simulink model "TPGCI_2"  (R2024a)
settings: Solver=FixedStepDiscrete  StartTime=0.0  StopTime=10.0  FixedStep=2e-5  RelTol=1e-3
undefined symbols (not defined in the file): DiscIntNeverNeededParam
libraries: slpidlib x3
settings Model: Creator=mahes  LastModifiedBy=mahes
settings OptimizationCC: DefaultParameterBehavior=Inlined  UseDivisionForNetSlopeComputation=on  GainParamInheritBuiltInType=on  UseFloatMulNetSlope=on  InlineInvariantSignals=on  PassReuseOutputArgsAs=Individual arguments  ZeroExternalMemoryAtStartup=off  ZeroInternalMemoryAtStartup=off  NoFixptDivByZeroProtection=on  EfficientFloat2IntCast=on  LifeSpan=1  OptimizeBlockOrder=speed  DifferentSizesBufferReuse=on  EfficientTunableParamExpr=on
settings DebuggingCC: ParameterTunabilityLossMsg=error
settings HardwareCC: ProdBitPerPointer=32  ProdBitPerSizeT=32  ProdBitPerPtrDiffT=32  ProdLargestAtomicInteger=Long  ProdLargestAtomicFloat=Double  ProdWordSize=32  ProdLongLongMode=on  ProdHWDeviceType=ARM Compatible->ARM Cortex-M
settings SFSimCC: MATLABDynamicMemAlloc=off
settings RTWCC: Description=Embedded Coder  SystemTargetFile=ert.tlc  TemplateMakefile=ert_default_tmf
settings CodeAppCC: ForceParamTrailComments=on  IgnoreCustomStorageClasses=off  OperatorAnnotations=on  SimulinkDataObjDesc=on  SFDataObjDesc=on  CustomSymbolStrGlobalVar=rt$N$M  CustomSymbolStrType=$N$M  CustomSymbolStrFcn=$N$M$F  CustomSymbolStrMacro=$N$M  InsertBlockDesc=on
settings ERTTargetCC: TargetLangStandard=C99 (ISO)  GenerateSampleERTMain=on  IncludeMdlTerminateFcn=off  CombineSignalStateStructs=on  SupportAbsoluteTime=off  SupportComplex=off  SupportNonInlinedSFcns=on  InlinedParameterPlacement=NonHierarchical  ERTCustomFileTemplate=example_file_process.tlc  ERTFilePackagingFormat=CompactWithDataFile

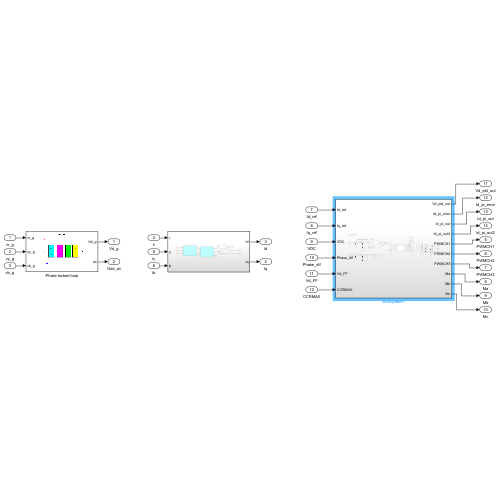
[thumbnail: Simulink's stored preview of the top-level diagram]
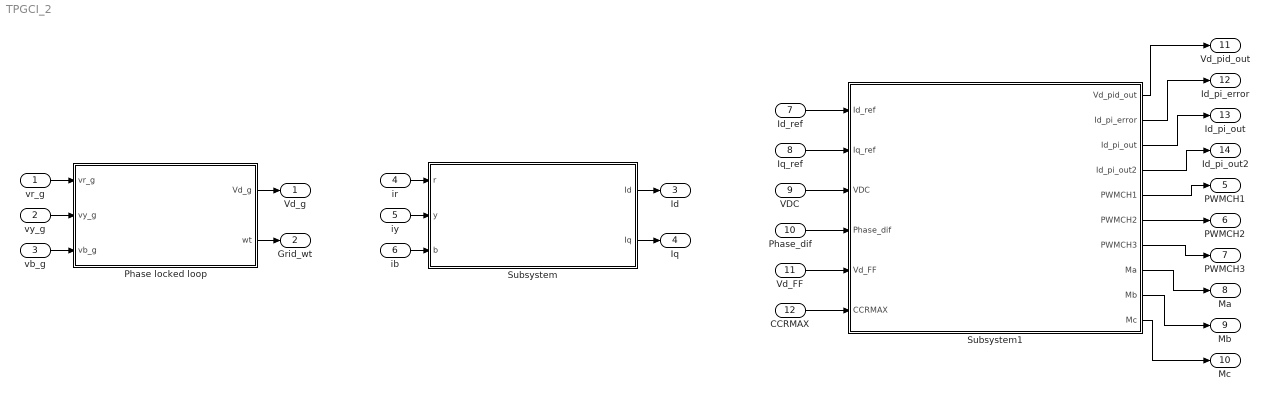
== system TPGCI_2 ==
  vr_g : Inport
  vy_g : Inport  Port=2
  vb_g : Inport  Port=3
  ir : Inport  Port=4
  iy : Inport  Port=5
  ib : Inport  Port=6
  Id_ref : Inport  Port=7
  Iq_ref : Inport  Port=8
  VDC : Inport  Port=9
  Phase_dif : Inport  Port=10
  Vd_FF : Inport  Port=11
  CCRMAX : Inport  Port=12
  Phase locked loop : Subsystem
      mask Display: image('abc_to_dq_pll_icon.png', [0,0,0,0,95,95]);
  Subsystem : Subsystem
  Subsystem1 : Subsystem
  Vd_g : Outport
  Grid_wt : Outport  Port=2
  Id : Outport  Port=3
  Iq : Outport  Port=4
  PWMCH1 : Outport  Port=5
  PWMCH2 : Outport  Port=6
  PWMCH3 : Outport  Port=7
  Ma : Outport  Port=8
  Mb : Outport  Port=9
  Mc : Outport  Port=10
  Vd_pid_out : Outport  Port=11
  Id_pi_error : Outport  Port=12
  Id_pi_out : Outport  Port=13
  Id_pi_out2 : Outport  Port=14
  wires:
  Iq_ref/1 -> Subsystem1/2(Iq_ref)
  Vd_FF/1 -> Subsystem1/5(Vd_FF)
  Subsystem/1(Id) -> Id/1
  VDC/1 -> Subsystem1/3(VDC)
  vy_g/1 -> Phase locked loop/2(vy_g)
  Phase locked loop/2(wt) -> Grid_wt/1
  ir/1 -> Subsystem/1(r)
  ib/1 -> Subsystem/3(b)
  vb_g/1 -> Phase locked loop/3(vb_g)
  Phase_dif/1 -> Subsystem1/4(Phase_dif)
  iy/1 -> Subsystem/2(y)
  Id_ref/1 -> Subsystem1/1(Id_ref)
  vr_g/1 -> Phase locked loop/1(vr_g)
  Subsystem/2(Iq) -> Iq/1
  Phase locked loop/1(Vd_g) -> Vd_g/1
  CCRMAX/1 -> Subsystem1/6(CCRMAX)
  Subsystem1/1(Vd_pid_out) -> Vd_pid_out/1
  Subsystem1/2(Id_pi_error) -> Id_pi_error/1
  Subsystem1/3(Id_pi_out) -> Id_pi_out/1
  Subsystem1/4(Id_pi_out2) -> Id_pi_out2/1
  Subsystem1/5(PWMCH1) -> PWMCH1/1
  Subsystem1/6(PWMCH2) -> PWMCH2/1
  Subsystem1/7(PWMCH3) -> PWMCH3/1
  Subsystem1/8(Ma) -> Ma/1
  Subsystem1/9(Mb) -> Mb/1
  Subsystem1/10(Mc) -> Mc/1

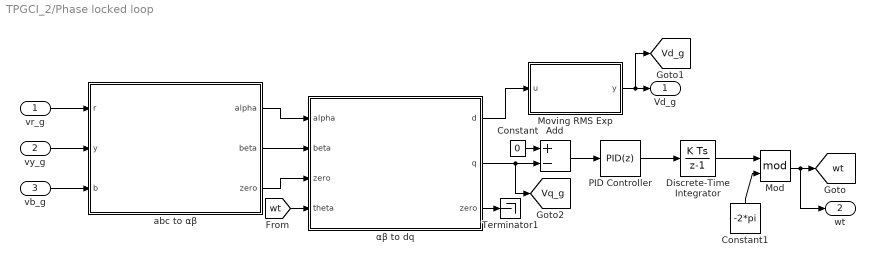
== system TPGCI_2/Phase locked loop ==
  vr_g : Inport
  vy_g : Inport  Port=2
  vb_g : Inport  Port=3
  Add : Sum  Inputs=+-
  Constant : Constant  Value=0
  Constant1 : Constant  Value=-2*pi
  Discrete-Time Integrator : DiscreteIntegrator  SampleTime=2e-5  ICPrevOutput=DiscIntNeverNeededParam  ICPrevScaledInput=DiscIntNeverNeededParam
  Mod : Math  Operator=mod
  Moving RMS Exp : MATLAB Function  TreatAsAtomicUnit=on
  PID Controller : slpidlib/PID Controller  Controller=PID  Form=Parallel  TimeDomain=Discrete-time  UseExternalTs=off  SampleTime=2e-5  IntegratorMethod=Forward Euler  FilterMethod=Forward Euler  ControllerParametersSource=internal  P=10  I=1000  UseKiTs=off  D=0  UseExternalDerivativeSource=off  N=100  UseFilter=on  TunerSelectOption=Transfer Function Based (PID Tuner App)  InitialConditionSource=internal  InitialConditionForIntegrator=0  InitialConditionForFilter=0  DifferentiatorICPrevScaledInput=0  ExternalReset=none  TrackingMode=off  Kt=1  LimitOutput=off  SatLimitsSource=internal  UpperSaturationLimit=inf  LowerSaturationLimit=-inf  LinearizeAsGain=on  AntiWindupMode=none  Kb=1  LimitIntegrator=off  UpperIntegratorSaturationLimit=inf  LowerIntegratorSaturationLimit=-inf  POutMin=[]  POutMax=[]  IOutMin=[]  IOutMax=[]  DOutMin=[]  DOutMax=[]  NOutMin=[]  NOutMax=[]  SumOutMin=[]  SumOutMax=[]  SaturationOutMin=[]  SaturationOutMax=[]  PParamMin=[]  PParamMax=[]  IParamMin=[]  IParamMax=[]  DParamMin=[]  DParamMax=[]  NParamMin=[]  NParamMax=[]  KbParamMin=[]  KbParamMax=[]  KtParamMin=[]  KtParamMax=[]  KbOutMin=[]  KbOutMax=[]  KtOutMin=[]  KtOutMax=[]  IntegratorOutMin=[]  IntegratorOutMax=[]  FilterOutMin=[]  FilterOutMax=[]  SumI1OutMin=[]  SumI1OutMax=[]  SumI2OutMin=[]  SumI2OutMax=[]  SumI3OutMin=[]  SumI3OutMax=[]  SumI4OutMin=[]  SumI4OutMax=[]  SumDOutMin=[]  SumDOutMax=[]  DifferentiatorOutMin=[]  DifferentiatorOutMax=[]  FilterDiffOutCoefMin=[]  FilterDiffOutCoefMax=[]  ReciprocalOutMin=[]  ReciprocalOutMax=[]  SumDenOutMin=[]  SumDenOutMax=[]  SumNumOutMin=[]  SumNumOutMax=[]  DivideOutMin=[]  DivideOutMax=[]  UdiffTsProdOutMin=[]  UdiffTsProdOutMax=[]  NTsProdOutMin=[]  NTsProdOutMax=[]  UintegralTsProdOutMin=[]  UintegralTsProdOutMax=[]  UngainTsProdOutMin=[]  UngainTsProdOutMax=[]  ClampingZeroOutDataTypeStr=Inherit: Inherit via back propagation  ClampingZeroOutMin=[]  ClampingZeroOutMax=[]  FilterDenConstantOutDataTypeStr=Inherit: Inherit via back propagation  FilterDenConstantOutMin=[]  FilterDenConstantOutMax=[]  PCopyOutDataTypeStr=Inherit: Inherit via back propagation  PCopyOutMin=[]  PCopyOutMax=[]  NCopyOutDataTypeStr=Inherit: Inherit via back propagation  NCopyOutMin=[]  NCopyOutMax=[]  IntegratorContinuousStateAttributes=''  IntegratorStateMustResolveToSignalObject=off  IntegratorRTWStateStorageClass=Auto  FilterContinuousStateAttributes=''  FilterStateMustResolveToSignalObject=off  FilterRTWStateStorageClass=Auto  ParallelPVariant=InternalParameters  IdealPVariant=Disabled  IVariant=InternalParameters  DVariant=InternalParameters  IntegratorVariant=Discrete  SatVariant=Disabled  AWVariant=Passthrough  PCopyVariant=Disabled  TRVariant=Disabled  FdbkBlocksVariant=Forward  IdealPFdbkVariant=Disabled  SatFdbkVariant=Disabled  DerivativeFilterVariant=ForwardEulerFilter  NVariant=InternalParameters  NCopyVariant=Disabled  FilterICVariant=InternalICsFilter  IntegratorICVariant=InternalICs  ExternalResetVariant=Disabled  TRSumVariant=Passthrough  SumFdbkVariant=Disabled  SumVariant=Sum_PID  TsampFilterVariant=InternalTs  TsampNgainVariant=Passthrough  TsampIntegralVariant=Disabled_SignalSpec  ExternalSaturationOutDataTypeStr=Inherit: Same as second input  DerivativeSourceVariant=ErrorSignal
  Terminator1 : Terminator
  abc to αβ : MATLAB Function  TreatAsAtomicUnit=on
  αβ to dq : MATLAB Function  TreatAsAtomicUnit=on
  Vd_g : Outport
  wt : Outport  Port=2
  tag scope: Vd_g=global, Vq_g=global, wt=global
  wires:
  αβ to dq/3(zero) -> Terminator1/1
  abc to αβ/2(beta) -> αβ to dq/2(beta)
  αβ to dq/1(d) -> Moving RMS Exp/1(u)
  [wt] -> αβ to dq/4(theta)
  abc to αβ/1(alpha) -> αβ to dq/1(alpha)
  abc to αβ/3(zero) -> αβ to dq/3("zero ")
  Mod/1 -> wt/1, [wt]
  Discrete-Time Integrator/1 -> Mod/1
  Constant1/1 -> Mod/2
  Constant/1 -> Add/1
  αβ to dq/2(q) -> [Vq_g], Add/2
  PID Controller/1 -> Discrete-Time Integrator/1
  Add/1 -> PID Controller/1
  vy_g/1 -> abc to αβ/2(y)
  vb_g/1 -> abc to αβ/3(b)
  vr_g/1 -> abc to αβ/1(r)
  Moving RMS Exp/1(y) -> [Vd_g], Vd_g/1

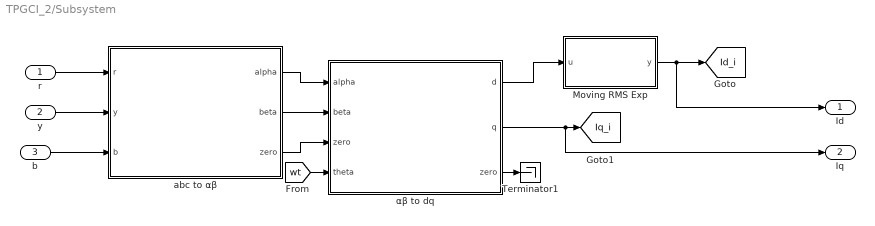
== system TPGCI_2/Subsystem ==
  r : Inport
  y : Inport  Port=2
  b : Inport  Port=3
  Moving RMS Exp : MATLAB Function  TreatAsAtomicUnit=on
  Terminator1 : Terminator
  abc to αβ : MATLAB Function  TreatAsAtomicUnit=on
  αβ to dq : MATLAB Function  TreatAsAtomicUnit=on
  Id : Outport
  Iq : Outport  Port=2
  tag scope: Id_i=global, Iq_i=global
  wires:
  abc to αβ/2(beta) -> αβ to dq/2(beta)
  αβ to dq/1(d) -> Moving RMS Exp/1(u)
  αβ to dq/2(q) -> Iq/1, [Iq_i]
  abc to αβ/1(alpha) -> αβ to dq/1(alpha)
  abc to αβ/3(zero) -> αβ to dq/3("zero ")
  αβ to dq/3(zero) -> Terminator1/1
  Moving RMS Exp/1(y) -> Id/1, [Id_i]
  [wt] -> αβ to dq/4(theta)
  y/1 -> abc to αβ/2(y)
  b/1 -> abc to αβ/3(b)
  r/1 -> abc to αβ/1(r)

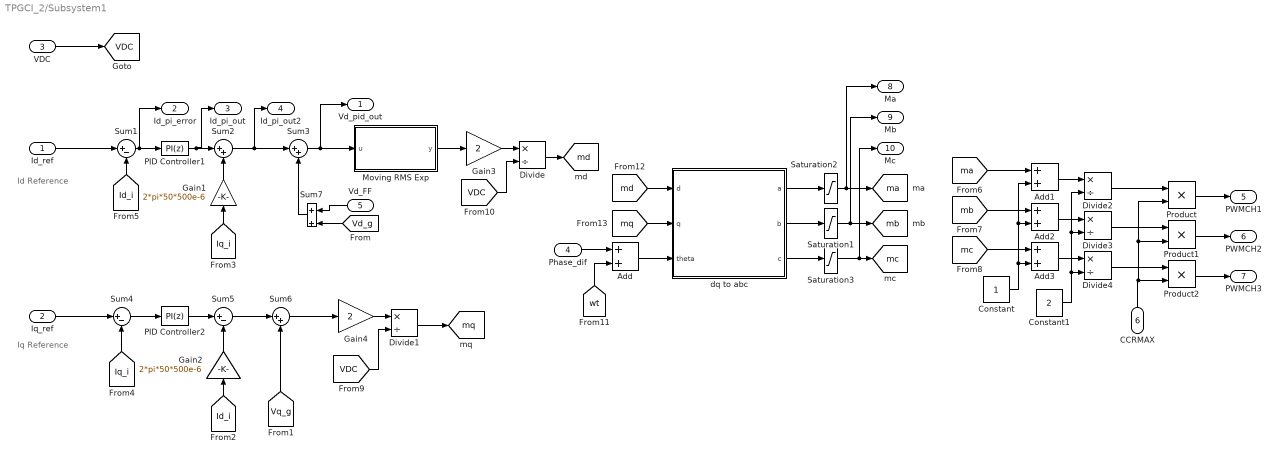
== system TPGCI_2/Subsystem1 ==
  note: Iq Reference
  note: Id Reference
  Id_ref : Inport
  Iq_ref : Inport  Port=2
  VDC : Inport  Port=3
  Phase_dif : Inport  Port=4
  Vd_FF : Inport  Port=5
  CCRMAX : Inport  Port=6
  Add{,1..3} (4 alike) : Sum
  Constant : Constant
  Constant1 : Constant  Value=2  VectorParams1D=off  SampleTime=-1
  Divide{,1..4} (5 alike) : Product  Inputs=*/
  Gain1 : Gain  Gain=2*pi*50*500e-6
  Gain2 : Gain  Gain=2*pi*50*500e-6
  Gain3 : Gain  Gain=2
  Gain4 : Gain  Gain=2
  Moving RMS Exp : MATLAB Function  TreatAsAtomicUnit=on
  PID Controller1 : slpidlib/PID Controller  Controller=PI  Form=Parallel  TimeDomain=Discrete-time  UseExternalTs=off  SampleTime=2e-5  IntegratorMethod=Forward Euler  FilterMethod=Forward Euler  ControllerParametersSource=internal  P=0.01  I=1  UseKiTs=off  D=0  UseExternalDerivativeSource=off  N=100  UseFilter=on  TunerSelectOption=Transfer Function Based (PID Tuner App)  InitialConditionSource=internal  InitialConditionForIntegrator=0  InitialConditionForFilter=0  DifferentiatorICPrevScaledInput=0  ExternalReset=none  TrackingMode=off  Kt=1  LimitOutput=on  SatLimitsSource=internal  UpperSaturationLimit=+10  LowerSaturationLimit=-10  LinearizeAsGain=on  AntiWindupMode=none  Kb=1  LimitIntegrator=on  UpperIntegratorSaturationLimit=+10  LowerIntegratorSaturationLimit=-10  RndMeth=Nearest  POutMin=[]  POutMax=[]  IOutMin=[]  IOutMax=[]  DOutMin=[]  DOutMax=[]  NOutMin=[]  NOutMax=[]  SumOutMin=[]  SumOutMax=[]  SaturationOutMin=[]  SaturationOutMax=[]  PParamMin=[]  PParamMax=[]  IParamMin=[]  IParamMax=[]  DParamMin=[]  DParamMax=[]  NParamMin=[]  NParamMax=[]  KbParamMin=[]  KbParamMax=[]  KtParamMin=[]  KtParamMax=[]  KbOutMin=[]  KbOutMax=[]  KtOutMin=[]  KtOutMax=[]  IntegratorOutMin=[]  IntegratorOutMax=[]  FilterOutMin=[]  FilterOutMax=[]  SumI1OutMin=[]  SumI1OutMax=[]  SumI2OutMin=[]  SumI2OutMax=[]  SumI3OutMin=[]  SumI3OutMax=[]  SumI4OutMin=[]  SumI4OutMax=[]  SumDOutMin=[]  SumDOutMax=[]  DifferentiatorOutMin=[]  DifferentiatorOutMax=[]  FilterDiffOutCoefMin=[]  FilterDiffOutCoefMax=[]  ReciprocalOutMin=[]  ReciprocalOutMax=[]  SumDenOutMin=[]  SumDenOutMax=[]  SumNumOutMin=[]  SumNumOutMax=[]  DivideOutMin=[]  DivideOutMax=[]  UdiffTsProdOutMin=[]  UdiffTsProdOutMax=[]  NTsProdOutMin=[]  NTsProdOutMax=[]  UintegralTsProdOutMin=[]  UintegralTsProdOutMax=[]  UngainTsProdOutMin=[]  UngainTsProdOutMax=[]  ClampingZeroOutDataTypeStr=Inherit: Inherit via back propagation  ClampingZeroOutMin=[]  ClampingZeroOutMax=[]  FilterDenConstantOutDataTypeStr=Inherit: Inherit via back propagation  FilterDenConstantOutMin=[]  FilterDenConstantOutMax=[]  PCopyOutDataTypeStr=Inherit: Inherit via back propagation  PCopyOutMin=[]  PCopyOutMax=[]  NCopyOutDataTypeStr=Inherit: Inherit via back propagation  NCopyOutMin=[]  NCopyOutMax=[]  IntegratorContinuousStateAttributes=''  IntegratorStateMustResolveToSignalObject=off  IntegratorRTWStateStorageClass=Auto  FilterContinuousStateAttributes=''  FilterStateMustResolveToSignalObject=off  FilterRTWStateStorageClass=Auto  ParallelPVariant=InternalParameters  IdealPVariant=Disabled  IVariant=InternalParameters  DVariant=Disabled  IntegratorVariant=Discrete  SatVariant=Enabled  AWVariant=Passthrough  PCopyVariant=Disabled  TRVariant=Disabled  FdbkBlocksVariant=Forward  IdealPFdbkVariant=Disabled  SatFdbkVariant=Disabled  DerivativeFilterVariant=Disabled  NVariant=Disabled  NCopyVariant=Disabled_SignalSpec  FilterICVariant=Disabled  IntegratorICVariant=InternalICs  ExternalResetVariant=Disabled  TRSumVariant=Passthrough  SumFdbkVariant=Disabled  SumVariant=Sum_PI  TsampFilterVariant=InternalTs  TsampNgainVariant=Passthrough  TsampIntegralVariant=Disabled_SignalSpec  ExternalSaturationOutDataTypeStr=Inherit: Same as second input  DerivativeSourceVariant=Disabled
  PID Controller2 : slpidlib/PID Controller  Controller=PI  Form=Parallel  TimeDomain=Discrete-time  UseExternalTs=off  SampleTime=2e-5  IntegratorMethod=Forward Euler  FilterMethod=Forward Euler  ControllerParametersSource=internal  P=0.01  I=1  UseKiTs=off  D=0  UseExternalDerivativeSource=off  N=100  UseFilter=on  TunerSelectOption=Transfer Function Based (PID Tuner App)  InitialConditionSource=internal  InitialConditionForIntegrator=0  InitialConditionForFilter=0  DifferentiatorICPrevScaledInput=0  ExternalReset=none  TrackingMode=off  Kt=1  LimitOutput=on  SatLimitsSource=internal  UpperSaturationLimit=10  LowerSaturationLimit=-10  LinearizeAsGain=on  AntiWindupMode=none  Kb=1  LimitIntegrator=on  UpperIntegratorSaturationLimit=10  LowerIntegratorSaturationLimit=-10  POutMin=[]  POutMax=[]  IOutMin=[]  IOutMax=[]  DOutMin=[]  DOutMax=[]  NOutMin=[]  NOutMax=[]  SumOutMin=[]  SumOutMax=[]  SaturationOutMin=[]  SaturationOutMax=[]  PParamMin=[]  PParamMax=[]  IParamMin=[]  IParamMax=[]  DParamMin=[]  DParamMax=[]  NParamMin=[]  NParamMax=[]  KbParamMin=[]  KbParamMax=[]  KtParamMin=[]  KtParamMax=[]  KbOutMin=[]  KbOutMax=[]  KtOutMin=[]  KtOutMax=[]  IntegratorOutMin=[]  IntegratorOutMax=[]  FilterOutMin=[]  FilterOutMax=[]  SumI1OutMin=[]  SumI1OutMax=[]  SumI2OutMin=[]  SumI2OutMax=[]  SumI3OutMin=[]  SumI3OutMax=[]  SumI4OutMin=[]  SumI4OutMax=[]  SumDOutMin=[]  SumDOutMax=[]  DifferentiatorOutMin=[]  DifferentiatorOutMax=[]  FilterDiffOutCoefMin=[]  FilterDiffOutCoefMax=[]  ReciprocalOutMin=[]  ReciprocalOutMax=[]  SumDenOutMin=[]  SumDenOutMax=[]  SumNumOutMin=[]  SumNumOutMax=[]  DivideOutMin=[]  DivideOutMax=[]  UdiffTsProdOutMin=[]  UdiffTsProdOutMax=[]  NTsProdOutMin=[]  NTsProdOutMax=[]  UintegralTsProdOutMin=[]  UintegralTsProdOutMax=[]  UngainTsProdOutMin=[]  UngainTsProdOutMax=[]  ClampingZeroOutDataTypeStr=Inherit: Inherit via back propagation  ClampingZeroOutMin=[]  ClampingZeroOutMax=[]  FilterDenConstantOutDataTypeStr=Inherit: Inherit via back propagation  FilterDenConstantOutMin=[]  FilterDenConstantOutMax=[]  PCopyOutDataTypeStr=Inherit: Inherit via back propagation  PCopyOutMin=[]  PCopyOutMax=[]  NCopyOutDataTypeStr=Inherit: Inherit via back propagation  NCopyOutMin=[]  NCopyOutMax=[]  IntegratorContinuousStateAttributes=''  IntegratorStateMustResolveToSignalObject=off  IntegratorRTWStateStorageClass=Auto  FilterContinuousStateAttributes=''  FilterStateMustResolveToSignalObject=off  FilterRTWStateStorageClass=Auto  ParallelPVariant=InternalParameters  IdealPVariant=Disabled  IVariant=InternalParameters  DVariant=Disabled  IntegratorVariant=Discrete  SatVariant=Enabled  AWVariant=Passthrough  PCopyVariant=Disabled  TRVariant=Disabled  FdbkBlocksVariant=Forward  IdealPFdbkVariant=Disabled  SatFdbkVariant=Disabled  DerivativeFilterVariant=Disabled  NVariant=Disabled  NCopyVariant=Disabled_SignalSpec  FilterICVariant=Disabled  IntegratorICVariant=InternalICs  ExternalResetVariant=Disabled  TRSumVariant=Passthrough  SumFdbkVariant=Disabled  SumVariant=Sum_PI  TsampFilterVariant=InternalTs  TsampNgainVariant=Passthrough  TsampIntegralVariant=Disabled_SignalSpec  ExternalSaturationOutDataTypeStr=Inherit: Same as second input  DerivativeSourceVariant=Disabled
  Product : Product
  Product1 : Product
  Product2 : Product
  Saturation1 : Saturate  UpperLimit=0.95  LowerLimit=-0.95
  Saturation2 : Saturate  UpperLimit=0.95  LowerLimit=-0.95
  Saturation3 : Saturate  UpperLimit=0.95  LowerLimit=-0.95
  Sum1 : Sum  Inputs=|+-
  Sum{2..3,6..7} (4 alike) : Sum  Inputs=|++
  Sum4 : Sum  Inputs=|+-
  Sum5 : Sum  Inputs=|+-
  dq to abc : MATLAB Function  TreatAsAtomicUnit=on
  Vd_pid_out : Outport
  Id_pi_error : Outport  Port=2
  Id_pi_out : Outport  Port=3
  Id_pi_out2 : Outport  Port=4
  PWMCH1 : Outport  Port=5
  PWMCH2 : Outport  Port=6
  PWMCH3 : Outport  Port=7
  Ma : Outport  Port=8
  Mb : Outport  Port=9
  Mc : Outport  Port=10
  tag scope: VDC=global, ma=global, mb=global, mc=global, md=global, mq=global
  wires:
  [Id_i] -> Gain2/1
  Sum4/1 -> PID Controller2/1
  Iq_ref/1 -> Sum4/1
  [Id_i] -> Sum1/2
  Sum2/1 -> Id_pi_out2/1, Sum3/1
  Sum3/1 -> Moving RMS Exp/1(u), Vd_pid_out/1
  PID Controller1/1 -> Id_pi_out/1, Sum2/1
  Gain1/1 -> Sum2/2
  Sum5/1 -> Sum6/1
  Sum1/1 -> Id_pi_error/1, PID Controller1/1
  PID Controller2/1 -> Sum5/1
  Gain2/1 -> Sum5/2
  [Vq_g] -> Sum6/2
  [Iq_i] -> Sum4/2
  [Iq_i] -> Gain1/1
  Id_ref/1 -> Sum1/1
  Add/1 -> dq to abc/3(theta)
  [wt] -> Add/2
  Phase_dif/1 -> Add/1
  Vd_FF/1 -> Sum7/1
  [Vd_g] -> Sum7/2
  Sum7/1 -> Sum3/2
  [VDC] -> Divide/2
  Divide/1 -> [md]
  Gain3/1 -> Divide/1
  Sum6/1 -> Gain4/1
  Divide1/1 -> [mq]
  Gain4/1 -> Divide1/1
  [VDC] -> Divide1/2
  [md] -> dq to abc/1(d)
  [mq] -> dq to abc/2(q)
  VDC/1 -> [VDC]
  Add1/1 -> Divide2/1
  [mc] -> Add3/1
  Constant/1 -> Add1/2, Add2/2, Add3/2
  [ma] -> Add1/1
  Add3/1 -> Divide4/1
  Add2/1 -> Divide3/1
  Divide4/1 -> Product2/1
  Divide3/1 -> Product1/1
  Constant1/1 -> Divide2/2, Divide3/2, Divide4/2
  CCRMAX/1 -> Product2/2, Product1/2, Product/2
  Product1/1 -> PWMCH2/1
  dq to abc/3(c) -> Saturation3/1
  dq to abc/1(a) -> Saturation2/1
  Saturation2/1 -> Ma/1, [ma]
  [mb] -> Add2/1
  Saturation3/1 -> Mc/1, [mc]
  Product2/1 -> PWMCH3/1
  Saturation1/1 -> Mb/1, [mb]
  Product/1 -> PWMCH1/1
  Divide2/1 -> Product/1
  dq to abc/2(b) -> Saturation1/1
  Moving RMS Exp/1(y) -> Gain3/1

== matlab function TPGCI_2/Phase locked loop/αβ to dq ==
  data: alpha input; d output; beta input; zero input; theta input; q output; zero output
function [d, q, zero] = alphabeta_to_dq(alpha, beta, zero, theta) 
%ALPHABETA_TO_DQ Converts αβ0 voltages to dq0 using Park Transform
% Inputs:
%   v_alpha - Alpha axis voltage
%   v_beta  - Beta axis voltage
%   v_zero  - Zero sequence voltage
%   theta   - Rotational angle (radians)
% Outputs:
%   v_d     - Direct axis voltage
%   v_q     - Quadrature axis voltage
%   v_zero  - Zero sequence voltage (unchanged)

    % Precompute sine and cosine for efficiency
    cos_theta = cos(theta);
    sin_theta = sin(theta);

    % Compute dq0 components
    d =  alpha * cos_theta + beta * sin_theta;
    q = -alpha * sin_theta + beta * cos_theta;
    % v_zero remains the same
end

== matlab function TPGCI_2/Phase locked loop/abc to αβ ==
  data: r input; alpha output; y input; b input; beta output; zero output
function [alpha, beta, zero] = abc_to_alphabeta(r, y, b) 
%#codegen
%ABC_TO_ALPHABETA Converts three-phase (ABC) voltages to αβ0 (Clark Transform)
% Inputs:
%   vr_g - Phase R voltage
%   vy_g - Phase Y voltage
%   vb_g - Phase B voltage
% Outputs:
%   v_alpha_g - Alpha axis voltage
%   v_beta_g  - Beta axis voltage
%   v_zero    - Zero sequence voltage
    % Precompute constants (avoiding divisions)
    k1 = 0.66666666667;  % 2/3
    k2 = 0.33333333333;  % 1/3
    k3 = 0.57735026919;  % sqrt(3)/3

    % Compute αβ0 components using direct arithmetic
    alpha = k1 * r - k2 * y - k2 * b;
    beta  = k3 * (y - b);
    zero    = k2 * (r + y + b);
end

== matlab function TPGCI_2/Phase locked loop/Moving RMS Exp ==
  data: y output; u input
function y = movingRMSExp(u)
    % y = movingRMSExp(u, alpha)
    % This function computes the exponential moving RMS of the input signal `u`.
    % The parameter `alpha` is the smoothing factor (0 < alpha <= 1).
    % A higher `alpha` gives more weight to recent values.

    % Persistent variables to maintain state between calls
    persistent rmsSquared

    % Initialize the exponential moving RMS on the first call
    if isempty(rmsSquared)
        rmsSquared = u^2; % Initialize with the square of the first value

    end

    % Update the exponentially weighted RMS squared
    rmsSquared = 0.001 * u^2 + (1 - 0.001) * rmsSquared;

    % Compute the RMS as the square root of the weighted sum
    y = sqrt(rmsSquared);
end

== matlab function TPGCI_2/Subsystem/abc to αβ ==
  data: r input; alpha output; y input; b input; beta output; zero output
function [alpha, beta, zero] = abc_to_alphabeta(r, y, b) 
%#codegen
%ABC_TO_ALPHABETA Converts three-phase (ABC) voltages to αβ0 (Clark Transform)
% Inputs:
%   vr_g - Phase R voltage
%   vy_g - Phase Y voltage
%   vb_g - Phase B voltage
% Outputs:
%   v_alpha_g - Alpha axis voltage
%   v_beta_g  - Beta axis voltage
%   v_zero    - Zero sequence voltage
    % Precompute constants (avoiding divisions)
    k1 = 0.66666666667;  % 2/3
    k2 = 0.33333333333;  % 1/3
    k3 = 0.57735026919;  % sqrt(3)/3

    % Compute αβ0 components using direct arithmetic
    alpha = k1 * r - k2 * y - k2 * b;
    beta  = k3 * (y - b);
    zero    = k2 * (r + y + b);
end

== matlab function TPGCI_2/Subsystem/αβ to dq ==
  data: alpha input; d output; beta input; zero input; theta input; q output; zero output
function [d, q, zero] = alphabeta_to_dq(alpha, beta, zero, theta) 
%ALPHABETA_TO_DQ Converts αβ0 voltages to dq0 using Park Transform
% Inputs:
%   v_alpha - Alpha axis voltage
%   v_beta  - Beta axis voltage
%   v_zero  - Zero sequence voltage
%   theta   - Rotational angle (radians)
% Outputs:
%   v_d     - Direct axis voltage
%   v_q     - Quadrature axis voltage
%   v_zero  - Zero sequence voltage (unchanged)

    % Precompute sine and cosine for efficiency
    cos_theta = cos(theta);
    sin_theta = sin(theta);

    % Compute dq0 components
    d =  alpha * cos_theta + beta * sin_theta;
    q = -alpha * sin_theta + beta * cos_theta;
    % v_zero remains the same
end

== matlab function TPGCI_2/Subsystem/Moving RMS Exp ==
  data: y output; u input
function y = movingRMSExp(u)
    % y = movingRMSExp(u, alpha)
    % This function computes the exponential moving RMS of the input signal `u`.
    % The parameter `alpha` is the smoothing factor (0 < alpha <= 1).
    % A higher `alpha` gives more weight to recent values.

    % Persistent variables to maintain state between calls
    persistent rmsSquared

    % Initialize the exponential moving RMS on the first call
    if isempty(rmsSquared)
        rmsSquared = u^2; % Initialize with the square of the first value
    end

    % Update the exponentially weighted RMS squared
    rmsSquared = 0.001 * u^2 + (1 - 0.001) * rmsSquared;

    % Compute the RMS as the square root of the weighted sum
    y = sqrt(rmsSquared);
end

== matlab function TPGCI_2/Subsystem1/dq to abc ==
  data: d input; a output; q input; theta input; b output; c output
function [a, b, c] = dq_to_abc(d, q, theta)
%#codegen
% Converts dq0 frame to abc (three-phase) frame.

% Constants (Precomputed for efficiency)
TWO_PI_OVER_3 = 2.094395102393195;  % 2*pi/3
NEG_TWO_PI_OVER_3 = -2.094395102393195; % -2*pi/3

% Precompute sine and cosine values for efficiency
cos_theta = cos(theta);
sin_theta = sin(theta);

% Compute phase voltages using precomputed angles
a = d * cos_theta - q * sin_theta;
b = d * cos(theta + NEG_TWO_PI_OVER_3) - q * sin(theta + NEG_TWO_PI_OVER_3);
c = d * cos(theta + TWO_PI_OVER_3) - q * sin(theta + TWO_PI_OVER_3);

end

== matlab function TPGCI_2/Subsystem1/Moving RMS Exp ==
  data: y output; u input
function y = movingRMSExp(u)
    % y = movingRMSExp(u, alpha)
    % This function computes the exponential moving RMS of the input signal `u`.
    % The parameter `alpha` is the smoothing factor (0 < alpha <= 1).
    % A higher `alpha` gives more weight to recent values.

    % Persistent variables to maintain state between calls
    persistent rmsSquared

    % Initialize the exponential moving RMS on the first call
    if isempty(rmsSquared)
        rmsSquared = u^2; % Initialize with the square of the first value
    end

    % Update the exponentially weighted RMS squared
    rmsSquared = 0.001 * u^2 + (1 - 0.001) * rmsSquared;

    % Compute the RMS as the square root of the weighted sum
    y = sqrt(rmsSquared);
end
